simulink model "jackvvi"  (R2020a)
settings: Solver=FixedStepAuto  StartTime=0.0  StopTime=10  FixedStep=1e-3  RelTol=1e-3  EnableMultiTasking=on
undefined symbols (not defined in the file): D1, D10, D12, D13, D2, D3, D5, D7, D9, PTA1, PTA2, PTB9, PTC17, PTC3, PTC4, PTD0, PTD1, PTD3
libraries: frdmk64flib x9
settings Model: ExtModeTrigDuration=5  Creator=ryanb  LastModifiedBy=jamescameron
settings OptimizationCC: EnhancedBackFolding=on  PassReuseOutputArgsAs=Individual arguments  ZeroExternalMemoryAtStartup=off  ZeroInternalMemoryAtStartup=off  MaxStackSize=64  OptimizeBlockOrder=speed  DifferentSizesBufferReuse=on  OptimizationCustomize=off  EfficientTunableParamExpr=on
settings DebuggingCC: ParameterTunabilityLossMsg=error  UnconnectedInputMsg=none  UnconnectedOutputMsg=none  UnconnectedLineMsg=none
settings HardwareCC: ProdBitPerPointer=32  ProdBitPerSizeT=32  ProdBitPerPtrDiffT=32  ProdLargestAtomicInteger=Long  ProdLargestAtomicFloat=Double  ProdWordSize=32  ProdHWDeviceType=ARM Compatible->ARM Cortex
settings ModelReferenceCC: EnableRefExpFcnMdlSchedulingChecks=off
settings SFSimCC: MATLABDynamicMemAlloc=off
settings RTWCC: SystemTargetFile=ert.tlc  HardwareBoard=NXP FRDM-K64F  TemplateMakefile=ert_default_tmf  Toolchain=GNU Tools for ARM Embedded Processors
settings CodeAppCC: ForceParamTrailComments=on  IgnoreCustomStorageClasses=off  OperatorAnnotations=on  SimulinkDataObjDesc=on  SFDataObjDesc=on  InsertBlockDesc=on
settings ERTTargetCC: ExtModeTransport=4  ExtModeMexFile=sendToCommService

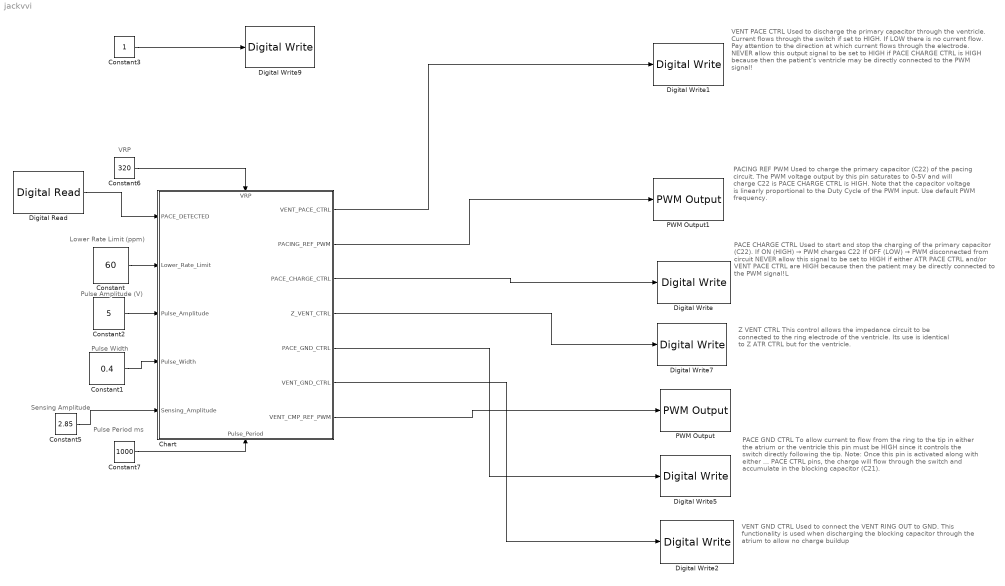
== system jackvvi ==
  note: Pulse Amplitude (V)
  note: Pulse Width
  note: Lower Rate Limit (ppm)
  note: Z VENT CTRL
      | This control allows the impedance circuit to be connected
      | to the ring electrode of the ventricle. Its use is identical to
      | Z ATR CTRL but for the ventricle.
  note: PACE GND CTRL
      | To allow current to flow from the ring to the tip in either the
      | atrium or the ventricle this pin must be HIGH since it controls
      | the switch directly following the tip.
      | Note: Once this pin is activated along with either ... PACE CTRL
      | pins, the charge will flow through the switch and accumulate in
      | the blocking capacitor (C21).
  note: PACING REF PWM
      | Used to charge the primary capacitor (C22) of the pacing circuit.
      | The PWM voltage output by this pin saturates to 0-5V and will
      | charge C22 is PACE CHARGE CTRL is HIGH.
      | Note that the capacitor voltage is linearly proportional to
      | the Duty Cycle of the PWM input. Use default PWM frequency.
  note: VENT GND CTRL
      | Used to connect the VENT RING OUT to GND. This functionality
      | is used when discharging the blocking capacitor through the
      | atrium to allow no charge buildup
  note: VENT PACE CTRL
      | Used to discharge the primary capacitor through the ventricle.
      | Current flows through the switch if set to HIGH. If LOW there is
      | no current flow. Pay attention to the direction at which current
      | flows through the electrode.
      | NEVER allow this output signal to be set to HIGH if
      | PACE CHARGE CTRL is HIGH because then the patient’s
      | ventricle may be directly connected to the PWM signal!
  note: PACE CHARGE CTRL
      | Used to start and stop the charging of the primary capacitor
      | (C22).
      | If ON (HIGH) → PWM charges C22
      | If OFF (LOW) → PWM disconnected from circuit
      | NEVER allow this signal to be set to HIGH if either
      | ATR PACE CTRL and/or VENT PACE CTRL are HIGH
      | because then the patient may be directly connected to the PWM
      | signal!L
  note: Sensing Amplitude
  note: VRP
  note: Pulse Period ms
  Chart : Stateflow chart  TreatAsAtomicUnit=on
      settings: PortSchema="{\"entries\":[{\"content\":{\"sides\":[{\"content\":{\"connectorIds\":[\"In4\",\"In5\",\"In6\",\"In7\",\"In3\"]},\"type\":\"ConnectorPlacement.EquallySpacedRectSide\",\"uuid\":\"72652cfb-0bb6-4258-a704-601e3c0b5d26\"},{\"content\":{\"connectorIds\":[\"Out1\",\"Out2\",\"Out3\",\"Out4\",\"Out5\",\"Out6\",\"Out7\"],\"side\":\"RIGHT\"},\"type\":\"ConnectorPlacement.EquallySpacedRectSide\",\"uuid\":\"51bd22d5-4d54-4764-997b-ab789807979b\"},{\"content\":{\"connectorIds\":[\"In2\"],\"side\":\"TOP\"},\"type\":\"ConnectorPlacement.EquallySpacedRectSide\",\"uuid\":\"b568f89c-a11f-4812-8dfe-f819792306b3\"},{\"content\":{\"connectorIds\":[\"In1\"],\"side\":\"BOTTOM\"},\"type\":\"ConnectorPlacement.EquallySpacedRectSide\",\"uuid\":\"a4e10e65-0031-4f7f-a850-f9aac3c2f857\"}]},\"type\":\"ConnectorPlacement.EquallySpacedConnector\",\"uuid\":\"bf9daf3b-2142-41fe-accd-96c7a2256776\"}],\"packageUris\":[\"http://schema.mathworks.com/mf0/Connector/19700101\"],\"version\":\"1.0\"}"
  Constant : Constant  Value=60
  Constant1 : Constant  Value=0.4
  Constant2 : Constant  Value=5
  Constant3 : Constant
  Constant5 : Constant  Value=2.85
  Constant6 : Constant  Value=320
  Constant7 : Constant  Value=1000
  Digital Read : frdmk64flib/Digital Read  Whichpin=PTC17 (D1)  SampleTime=-1
  Digital Write : frdmk64flib/Digital Write  Whichpin=PTB9 (D2)
  Digital Write1 : frdmk64flib/Digital Write  Whichpin=PTC4 (D9)
  Digital Write2 : frdmk64flib/Digital Write  Whichpin=PTD3 (D12)
  Digital Write5 : frdmk64flib/Digital Write  Whichpin=PTD0 (D10)
  Digital Write7 : frdmk64flib/Digital Write  Whichpin=PTC3 (D7)
  Digital Write9 : frdmk64flib/Digital Write  Whichpin=PTD1 (D13)
  PWM Output : frdmk64flib/PWM Output  Whichpin=PTA1 (D3)  InitialFrequency=2000  InitialDutyCycle=0
  PWM Output1 : frdmk64flib/PWM Output  Whichpin=PTA2 (D5)  InitialFrequency=2000  InitialDutyCycle=0
  wires:
  Chart/1(VENT_PACE_CTRL) -> Digital Write1/1
  Chart/2(PACING_REF_PWM) -> PWM Output1/1
  Chart/3(PACE_CHARGE_CTRL) -> Digital Write/1
  Chart/4(Z_VENT_CTRL) -> Digital Write7/1
  Chart/5(PACE_GND_CTRL) -> Digital Write5/1
  Chart/6(VENT_GND_CTRL) -> Digital Write2/1
  Constant2/1 -> Chart/6(Pulse_Amplitude)
  Constant1/1 -> Chart/7(Pulse_Width)
  Constant/1 -> Chart/5(Lower_Rate_Limit)
  Digital Read/1 -> Chart/4(PACE_DETECTED)
  Chart/7(VENT_CMP_REF_PWM) -> PWM Output/1
  Constant5/1 -> Chart/3(Sensing_Amplitude)
  Constant6/1 -> Chart/2(VRP)
  Constant7/1 -> Chart/1(Pulse_Period)
  Constant3/1 -> Digital Write9/1

== stateflow chart jackvvi/Chart ==
  state CHARGING
    entry:
    %%Charging C22
    PACING_REF_PWM = (Pulse_Amplitude/5.0)*100;
    VENT_CMP_REF_PWM = (Sensing_Amplitude/5)*100;
    VENT_PACE_CTRL = 0;
    PACE_CHARGE_CTRL = 1;
    %%Discharging Blocking Cap
    PACE_GND_CTRL = 0;
    Z_VENT_CTRL = 0;
    VENT_GND_CTRL = 1;
  state PACING
    entry:
    PACE_CHARGE_CTRL = 0;
    PACING_REF_PWM = (Pulse_Amplitude/5.0)*100;
    PACE_GND_CTRL = 1;
    Z_VENT_CTRL = 0;
    VENT_GND_CTRL = 0;
    VENT_PACE_CTRL = 1;
  (default) -> CHARGING
  (junction 28) -> PACING [order 2] : after(Pulse_Period - Pulse_Width - VRP,msec)[PACE_DETECTED == 0]
  (junction 28) -> CHARGING [order 1] : [PACE_DETECTED == true]
  CHARGING -> (junction 28) : [after(VRP,msec)]
  PACING -> CHARGING : %%Recharge Ready
      | [after(Pulse_Width, msec)]
  data: Pulse_Period input; VRP input; Sensing_Amplitude input; PACE_DETECTED input; VENT_PACE_CTRL output; PACING_REF_PWM output; PACE_CHARGE_CTRL output; Z_VENT_CTRL output; PACE_GND_CTRL output; VENT_GND_CTRL output; Lower_Rate_Limit input; Pulse_Amplitude input; Pulse_Width input; VENT_CMP_REF_PWM output
